simulink model "mainSim"  (Simulink 7.8)
settings: Solver=ode45  StartTime=0.0  StopTime=15  RelTol=1e-3
model workspace (MAT data in the model file):
  op_trim2 : opcond.OperatingReport (value not decoded)
values from neighbouring files (symbols this model uses):
  alt = h    [mainScript.m]
  defAilMax = 20*pi/180    (= 0.349065850399)    [mainScript.m]
  defElevMax = 25*pi/180    (= 0.436332312999)    [mainScript.m]
  defRudMax = 16*pi/180    (= 0.279252680319)    [mainScript.m]
  defThrotMax = 20    [mainScript.m]
  defTrims = [0*pi/180 -5*pi/180 0*pi/180 .5]    [mainScript.m]
  forcesReDimRefs = [Sref Sref Sref]    [mainScript.m]
  latCoeffRefs = [CY0 Cl0 Cn0]    [mainScript.m]
  latMatrix = [CYbeta CYbetaDot CYP CYR CYdeltaA CYdeltaR ... (first row only)    [mainScript.m]
  latNonDimRefs = [1 bref/(2*u0) bref/(2*u0)  bref/(2*u0) 1 1]    [mainScript.m]
  latStateRefs = [beta0 betaDot0 p0 q0 deltaA0 deltaR0]    [mainScript.m]
  longCoeffRefs = [-CD1 -CL0 CM1]    [mainScript.m]
  longMatrix = [CXu CXalpha CXalphaDot CXq CXdeltaE ... (first row only)    [mainScript.m]
  longNonDimRefs = [1/u0 1 cref/(2*u0) cref/(2*u0) 1]    [mainScript.m]
  longStateRefs = [u0 alpha0  alphaDot0 q0 deltaE0]    [mainScript.m]
  momentReDimRefs = [Sref*bref Sref*cref Sref*bref]    [mainScript.m]
  speed = v    [mainScript.m]
  Thrust = Tprop    [mainScript.m]
  Torque = QProp    [mainScript.m]
  V0 = [220 0 0]    [mainScript.m]
  Volt = V    [mainScript.m]
undefined symbols (not defined in the file or in its folder): Earth, WGS84
libraries: simulink x4, aerolibconvert2 x3, aerolibfltsims x2, aerolib6dof2 x1, aerolibatmos2 x1, aerolibtransform2 x1, aerolibasang x1, aerolibutil x1, aerolibanimutils x1
settings Model: Creator=mufasa  LastModifiedBy=atchase
settings DataIOCC: ExternalInput=getinputstruct(op_trim2)  InitialState=getstatestruct(op_trim2)  SignalLoggingSaveFormat=Dataset
settings GRTTargetCC: CombineOutputUpdateFcns=on

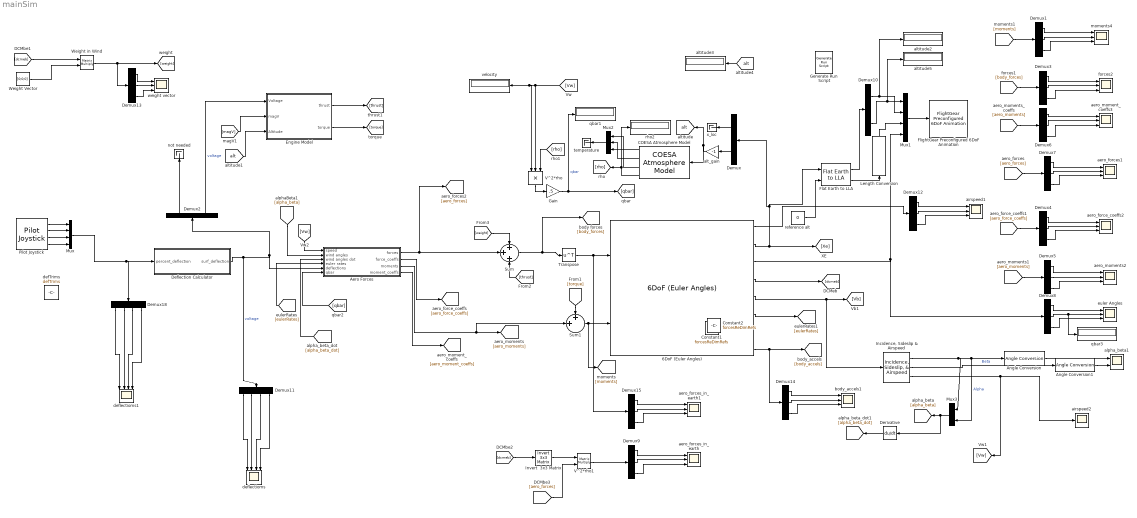
== system mainSim ==
  6DoF (Euler Angles) : aerolib6dof2/6DoF (Euler Angles)  units=English (Velocity in ft/s)  mtype=Fixed  rep=Quaternion  xme_0=X0  Vm_0=[V0(1) 0 0]  eul_0=[0 0 0]  pm_0=eulerRate0  mass_0=W  mass_e=0.5  mass_f=2.0  inertia=J  inertia_e=eye(3)  inertia_f=2*eye(3)  k_quat=1.0
  Aero Forces : Subsystem
  Angle Conversion : aerolibconvert2/Angle Conversion  IU=rad  OU=deg
  Angle Conversion1 : aerolibconvert2/Angle Conversion  IU=rad  OU=deg
  COESA Atmosphere Model : aerolibatmos2/COESA Atmosphere Model  units=English (Velocity in ft/s)  spec=1976 COESA-extended U.S. Standard Atmosphere  model=Profile  profile_var=High temperature  profile_percent=1%  profile_alt=5 km (16404 ft)  envelope_var=High temperature  envelope_percent=1%  action=Warning
  Constant1 : Constant  Value=forcesReDimRefs
  Constant2 : Constant  Value=forcesReDimRefs
  Deflection Calculator : Subsystem
  Demux : Demux  Outputs=[2 1]
  Demux{1,3..9,12..15} (12 alike) : Demux  Outputs=3
  Demux10 : Demux  Outputs=2
  Demux11 : Demux
  Demux18 : Demux
  Demux2 : Demux  Outputs=[3 1]
  Derivative : Derivative
  Engine Model : Subsystem
  Flat Earth to LLA : aerolibtransform2/Flat Earth to LLA  units=English  ptype=Earth (WGS84)  F=1/298.257223563  R=20925646.3255  LL0=[37 -121]  psi=0
  FlightGear Preconfigured 6DoF Animation : aerolibfltsims/FlightGear Preconfigured 6DoF Animation  xFlightGearVersion=v2.0  DestinationIpAddress=129.65.189.108  DestinationPort=5502  SampleTime=1/30
  Gain : Gain  Gain=.5
  Generate Run Script : aerolibfltsims/Generate Run Script  OutputFileName=runfg.bat  FlightGearBaseDirectory=C:\Program Files\FlightGear  GeometryModelName=c172p  DestinationPort=5502  AirportId=KSFO  RunwayId=10L  InitialAltitude=7224  InitialHeading=113  OffsetDistance=4.72  OffsetAzimuth=0  GenerateFile=off
  "Incidence, Sideslip & Airspeed" : aerolibasang/Incidence, Sideslip, & Airspeed
  Invert  3x3 Matrix : aerolibutil/Invert  3x3 Matrix
  Length Conversion : aerolibconvert2/Length Conversion  IU=ft  OU=m
  Mux : Mux
  Mux1 : Mux  Inputs=[1 1 1 3]
  Mux2 : Mux  Inputs=3
  Mux3 : Mux  Inputs=2
  Pilot Joystick : aerolibanimutils/Pilot Joystick  JoystickID=Joystick1  OutputConfiguration=FourAxis  SampleTime=1/30
  Sum : Sum  Inputs=+++
  Sum1 : Sum  Inputs=++|
  Transpose : Math  Operator=transpose  SaturateOnIntegerOverflow=on
  V^2*rho : Product  Inputs=3  RndMeth=Zero
  V^2*rho1 : Product  Multiplication=Matrix(*)  RndMeth=Zero
  Weight Vector : Constant  Value=[0;0;0]  VectorParams1D=off
  Weight in Wind : Product  Multiplication=Matrix(*)  RndMeth=Zero
  aero_force_coeffs2 : Scope  NumInputPorts=3
      settings: TimeRange=30  YMin=-0.5~-1~-4  YMax=0.5~1~4  SaveName=ScopeData3
  aero_forces1 : Scope  NumInputPorts=3
      settings: TimeRange=30  YMin=-2300~-1~-5000  YMax=-200~1~65000  SaveName=ScopeData4
  aero_forces_in_earth : Scope  NumInputPorts=3
      settings: TimeRange=100  YMin=-650~-1~-3515  YMax=-617.5~1~-3425  SaveName=ScopeData6
  aero_forces_in_earth1 : Scope  NumInputPorts=3
      settings: TimeRange=30  YMin=-650~-1~-3515  YMax=-617.5~1~-3425  SaveName=ScopeData11
  aero_moment_coeffs3 : Scope  NumInputPorts=3
      settings: TimeRange=30  YMin=0.309~-1~-1  YMax=0.332~1~1  SaveName=ScopeData5
  aero_moments2 : Scope  NumInputPorts=3
      settings: TimeRange=100  YMin=-1~-1~2517.5  YMax=1~1~2782.5  SaveName=ScopeData2
  airspeed1 : Scope  NumInputPorts=3
      settings: TimeRange=5  YMin=196.4~-1~-17.05  YMax=197.2~1~-16.25  SaveName=ScopeData13
  airspeed2 : Scope
      settings: TimeRange=5  YMin=213.55  YMax=213.69  SaveName=ScopeData17
  alpha_beta1 : Scope  NumInputPorts=2
      settings: TimeRange=25  YMin=-60~-1  YMax=60~1  SaveName=ScopeData16
  alt_gain : Gain  Gain=-1
  altitude2 : Display
  altitude3 : Display
  altitude5 : Display
  body_accels1 : Scope  NumInputPorts=3
      settings: TimeRange=100  YMin=-0.17~-1~-0.005  YMax=-0.156~1~0.095  SaveName=ScopeData10
  defTrims : Constant  Value=defTrims
  deflectioms : Scope  NumInputPorts=4
      settings: YMin=0.0025908~-1.1~-1~19  YMax=0.00286352~1.1~1~21  SaveName=ScopeData7
  deflectioms1 : Scope  NumInputPorts=4
      settings: TimeRange=5  YMin=-0.8~-0.01~-0.08~-1  YMax=0.6~0.08~0~1  SaveName=ScopeData14
  euler Angles : Scope  NumInputPorts=3
      settings: TimeRange=100  YMin=1.5708~2.75e-017~0.125  YMax=1.5708~8.5e-017~0.4  SaveName=ScopeData8
  forces2 : Scope  NumInputPorts=3
      settings: TimeRange=30  YMin=-119.5~-1~310.5  YMax=-116.5~1~310.69
  moments4 : Scope  NumInputPorts=3
      settings: TimeRange=30  YMin=0.309~-1~-1  YMax=0.332~1~1
  not needed : Terminator
  qbar1 : Display
  qbar3 : Display
  reference alt : Constant  Value=0
  rho2 : Display
  temperature : Terminator
  velocity : Display
  weight vector : Scope  NumInputPorts=3
      settings: TimeRange=5  YMin=-1~2517.5~5.58997e-013  YMax=1~2782.5~6.17839e-013  SaveName=ScopeData9
  x_loc : Terminator
  tag scope: alt=global
  wires:
  Pilot Joystick/1 -> Mux/1
  Pilot Joystick/2 -> Mux/2
  Pilot Joystick/3 -> Mux/3
  Pilot Joystick/4 -> Mux/4
  Deflection Calculator/1(surf_deflection) -> Demux11/1, Demux2/1, Aero Forces/5(deflections)  "voltage"
  Demux/1 -> x_loc/1
  Demux/2 -> alt_gain/1
  V^2*rho/1 -> Gain/1
  Mux/1 -> Demux18/1, Deflection Calculator/1(percent_deflection)
  reference alt/1 -> Flat Earth to LLA/2
  Mux1/1 -> FlightGear Preconfigured 6DoF Animation/1
  Flat Earth to LLA/1 -> Demux10/1
  alt_gain/1 -> [alt], COESA Atmosphere Model/1
  Demux11/1 -> deflectioms/1
  Demux11/2 -> deflectioms/2
  Demux11/3 -> deflectioms/3
  Demux11/4 -> deflectioms/4
  COESA Atmosphere Model/4 -> [rho], rho2/1
  Demux2/2 -> Engine Model/1(Voltage)  "voltage"
  Demux2/1 -> not needed/1
  [alt] -> Engine Model/3(Altitude)
  [magV] -> Engine Model/2(magV)
  Engine Model/1(thrust) -> [thrust]
  Engine Model/2(torque) -> [torque]
  Gain/1 -> [qbar], qbar1/1  "qbar"
  [alt] -> altitude3/1
  Sum1/1 -> 6DoF (Euler Angles)/2, [moments]
  [torque] -> Sum1/1
  [thrust] -> Sum/3
  Flat Earth to LLA/2 -> Length Conversion/1
  6DoF (Euler Angles)/2 -> Flat Earth to LLA/1, Demux/1, [Xe]
  6DoF (Euler Angles)/4 -> [dcmeb]
  [dcmeb] -> Weight in Wind/1
  Weight Vector/1 -> Weight in Wind/2
  Weight in Wind/1 -> [weight], Demux13/1
  Demux13/1 -> weight vector/1
  Demux13/2 -> weight vector/2
  Demux13/3 -> weight vector/3
  6DoF (Euler Angles)/3 -> Mux1/4, Demux8/1
  Length Conversion/1 -> Mux1/3
  Demux10/2 -> Mux1/1, altitude5/1
  Demux10/1 -> Mux1/2, altitude2/1
  6DoF (Euler Angles)/5 -> [Vb], "Incidence, Sideslip & Airspeed"/1
  Sum/1 -> [body_forces], Transpose/1
  6DoF (Euler Angles)/8 -> [body_accels], Demux14/1
  [qbar] -> Aero Forces/6(qbar)
  6DoF (Euler Angles)/6 -> [eulerRates]
  [eulerRates] -> Aero Forces/4(euler rates)
  [alpha_beta_dot] -> Aero Forces/3(wind angles dot)
  [alpha_beta] -> Aero Forces/2(wind angles)
  [Vw] -> Aero Forces/1(speed)
  COESA Atmosphere Model/1 -> Mux2/1
  COESA Atmosphere Model/2 -> Mux2/2
  COESA Atmosphere Model/3 -> Mux2/3
  Mux2/1 -> temperature/1
  Demux18/1 -> deflectioms1/1
  Demux18/2 -> deflectioms1/2
  Demux18/3 -> deflectioms1/3
  Demux18/4 -> deflectioms1/4
  Demux1/2 -> moments4/2
  Demux1/3 -> moments4/3
  Demux1/1 -> moments4/1
  [moments] -> Demux1/1
  [weight] -> Sum/1
  Demux3/2 -> forces2/2
  Demux3/3 -> forces2/3
  Demux3/1 -> forces2/1
  [body_forces] -> Demux3/1
  Demux4/2 -> aero_force_coeffs2/2
  Demux4/3 -> aero_force_coeffs2/3
  Demux4/1 -> aero_force_coeffs2/1
  [aero_force_coeffs] -> Demux4/1
  Demux5/2 -> aero_moments2/2
  Demux5/3 -> aero_moments2/3
  Demux5/1 -> aero_moments2/1
  [aero_moments] -> Demux5/1
  Demux6/2 -> aero_moment_coeffs3/2
  Demux6/3 -> aero_moment_coeffs3/3
  Demux6/1 -> aero_moment_coeffs3/1
  [aero_moments] -> Demux6/1
  Demux7/2 -> aero_forces1/2
  Demux7/3 -> aero_forces1/3
  Demux7/1 -> aero_forces1/1
  [aero_forces] -> Demux7/1
  Demux12/2 -> airspeed1/2
  Demux12/3 -> airspeed1/3
  Demux12/1 -> airspeed1/1
  6DoF (Euler Angles)/1 -> Demux12/1
  "Incidence, Sideslip & Airspeed"/1 -> Mux3/1, Mux3/2, Angle Conversion/1  "Alpha"
  "Incidence, Sideslip & Airspeed"/2 -> Angle Conversion1/1  "Beta"
  Mux3/1 -> [alpha_beta], Derivative/1
  Derivative/1 -> [alpha_beta_dot]
  "Incidence, Sideslip & Airspeed"/3 -> airspeed2/1, [Vw]
  [Vw] -> V^2*rho/2, velocity/1, V^2*rho/1
  [rho] -> V^2*rho/3
  Angle Conversion/1 -> alpha_beta1/1
  Angle Conversion1/1 -> alpha_beta1/2
  Demux8/2 -> euler Angles/2, qbar3/1
  Demux8/3 -> euler Angles/3
  Demux8/1 -> euler Angles/1
  [dcmeb] -> Invert  3x3 Matrix/1
  Invert  3x3 Matrix/1 -> V^2*rho1/1
  [aero_forces] -> V^2*rho1/2
  Demux9/2 -> aero_forces_in_earth/2
  Demux9/3 -> aero_forces_in_earth/3
  Demux9/1 -> aero_forces_in_earth/1
  V^2*rho1/1 -> Demux9/1
  Demux14/2 -> body_accels1/2
  Demux14/3 -> body_accels1/3
  Demux14/1 -> body_accels1/1
  Demux15/2 -> aero_forces_in_earth1/2
  Demux15/3 -> aero_forces_in_earth1/3
  Demux15/1 -> aero_forces_in_earth1/1
  Aero Forces/2(force_coeffs) -> [aero_force_coeffs]
  Aero Forces/4(moment_coeffs) -> [aero_moment_coeffs]
  Aero Forces/1(forces) -> [aero_forces], Sum/2
  Aero Forces/3(moments) -> [aero_moments], Sum1/2
  Transpose/1 -> 6DoF (Euler Angles)/1, Demux15/1

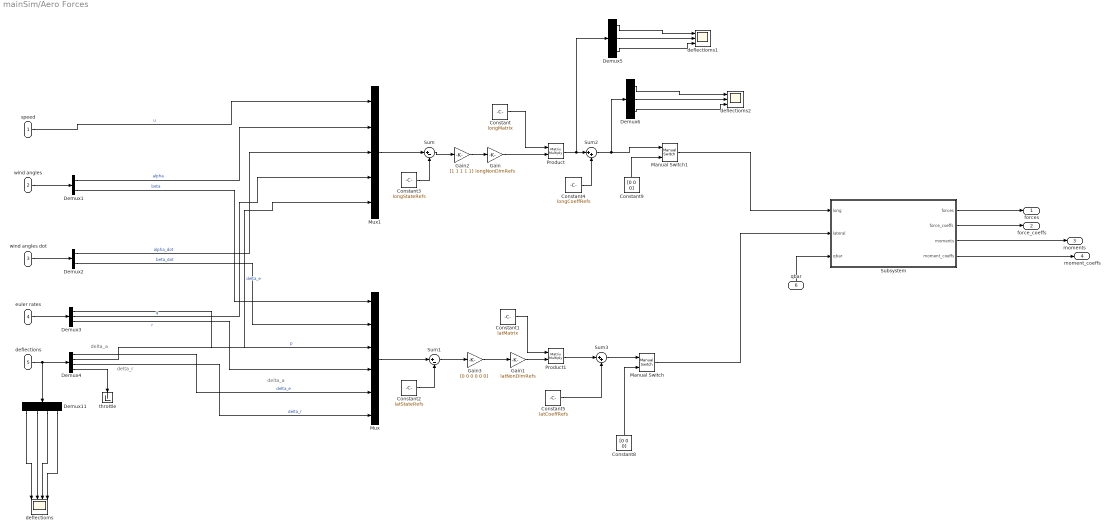
== system mainSim/Aero Forces ==
  note: delta_a
  note: delta_r
  note: delta_a
  speed : Inport
  wind angles : Inport  Port=2
  wind angles dot : Inport  Port=3
  euler rates : Inport  Port=4
  deflections : Inport  Port=5
  qbar : Inport  Port=6
  Constant : Constant  Value=longMatrix
  Constant1 : Constant  Value=latMatrix
  Constant2 : Constant  Value=latStateRefs
  Constant3 : Constant  Value=longStateRefs
  Constant4 : Constant  Value=longCoeffRefs
  Constant5 : Constant  Value=latCoeffRefs
  Constant8 : Constant  Value=[0 0 0]
  Constant9 : Constant  Value=[0 0 0]
  Demux1 : Demux  Outputs=2
  Demux11 : Demux
  Demux2 : Demux  Outputs=2
  Demux3 : Demux  Outputs=3
  Demux4 : Demux
  Demux5 : Demux  Outputs=3
  Demux6 : Demux  Outputs=3
  Gain : Gain  Gain=longNonDimRefs
  Gain1 : Gain  Gain=latNonDimRefs
  Gain2 : Gain  Gain=[1 1 1 1 1]
  Gain3 : Gain  Gain=[0 0 0 0 0 0]
  Manual Switch : simulink/Signal Routing/Manual Switch  sw=1  action=0  varsize=off
  Manual Switch1 : simulink/Signal Routing/Manual Switch  sw=1  action=0  varsize=off
  Mux : Mux  Inputs=6
  Mux1 : Mux  Inputs=5
  Product : Product  Multiplication=Matrix(*)  RndMeth=Zero
  Product1 : Product  Multiplication=Matrix(*)  RndMeth=Zero
  Subsystem : Subsystem
  Sum : Sum  Inputs=|+-
  Sum1 : Sum  Inputs=|+-
  Sum2 : Sum  Inputs=|++
  Sum3 : Sum  Inputs=|++
  deflectioms : Scope  NumInputPorts=4
      settings: YMin=0.0025908~-1.1~-1~19  YMax=0.00286352~1.1~1~21  SaveName=ScopeData15
  deflectioms1 : Scope  NumInputPorts=3
      settings: TimeRange=200  YMin=0.0025908~-1.1~-1  YMax=0.00286352~1.1~1  SaveName=ScopeData12
  deflectioms2 : Scope  NumInputPorts=3
      settings: TimeRange=200  YMin=0.0025908~-1.1~-1  YMax=0.00286352~1.1~1  SaveName=ScopeData18
  throttle : Terminator
  forces : Outport
  force_coeffs : Outport  Port=2
  moments : Outport  Port=3
  moment_coeffs : Outport  Port=4
  wires:
  speed/1 -> Mux1/1  "u"
  wind angles/1 -> Demux1/1
  wind angles dot/1 -> Demux2/1
  euler rates/1 -> Demux3/1
  deflections/1 -> Demux11/1, Demux4/1
  Demux1/1 -> Mux1/2  "alpha"
  Demux2/1 -> Mux1/3  "alpha_dot"
  Demux11/1 -> deflectioms/1
  Demux11/2 -> deflectioms/2
  Demux11/3 -> deflectioms/3
  Demux11/4 -> deflectioms/4
  Demux4/4 -> throttle/1
  Demux4/2 -> Mux1/5  "delta_e"
  Demux3/2 -> Mux1/4  "q"
  Demux1/2 -> Mux/1  "beta"
  Demux2/2 -> Mux/2  "beta_dot"
  Demux3/1 -> Mux/3  "p"
  Demux3/3 -> Mux/4  "r"
  Demux4/3 -> Mux/6  "delta_r"
  Demux4/1 -> Mux/5  "delta_e"
  Constant/1 -> Product/1
  Constant1/1 -> Product1/1
  Mux1/1 -> Sum/1
  Mux/1 -> Sum1/1
  Sum1/1 -> Gain3/1
  Constant2/1 -> Sum1/2
  Constant3/1 -> Sum/2
  Sum/1 -> Gain2/1
  Product/1 -> Sum2/1, Demux5/1
  Product1/1 -> Sum3/1
  Constant4/1 -> Sum2/2
  Constant5/1 -> Sum3/2
  Gain/1 -> Product/2
  Gain1/1 -> Product1/2
  Sum2/1 -> Manual Switch1/1, Demux6/1
  Sum3/1 -> Manual Switch/1
  Constant8/1 -> Manual Switch/2
  Constant9/1 -> Manual Switch1/2
  Manual Switch1/1 -> Subsystem/1(long)
  Manual Switch/1 -> Subsystem/2(lateral)
  qbar/1 -> Subsystem/3(qbar)
  Subsystem/1(forces) -> forces/1
  Subsystem/2(force_coeffs) -> force_coeffs/1
  Demux5/1 -> deflectioms1/1
  Demux5/2 -> deflectioms1/2
  Demux5/3 -> deflectioms1/3
  Demux6/1 -> deflectioms2/1
  Demux6/2 -> deflectioms2/2
  Demux6/3 -> deflectioms2/3
  Gain2/1 -> Gain/1
  Gain3/1 -> Gain1/1
  Subsystem/3(moments) -> moments/1
  Subsystem/4(moment_coeffs) -> moment_coeffs/1

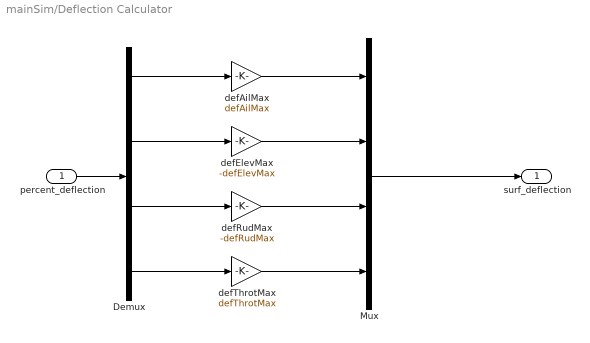
== system mainSim/Deflection Calculator ==
  percent_deflection : Inport
  Demux : Demux
  Mux : Mux
  defAilMax : Gain  Gain=defAilMax
  defElevMax : Gain  Gain=-defElevMax
  defRudMax : Gain  Gain=-defRudMax
  defThrotMax : Gain  Gain=defThrotMax
  surf_deflection : Outport
  wires:
  percent_deflection/1 -> Demux/1
  Demux/1 -> defAilMax/1
  Demux/2 -> defElevMax/1
  Demux/3 -> defRudMax/1
  Demux/4 -> defThrotMax/1
  Mux/1 -> surf_deflection/1
  defAilMax/1 -> Mux/1
  defElevMax/1 -> Mux/2
  defRudMax/1 -> Mux/3
  defThrotMax/1 -> Mux/4

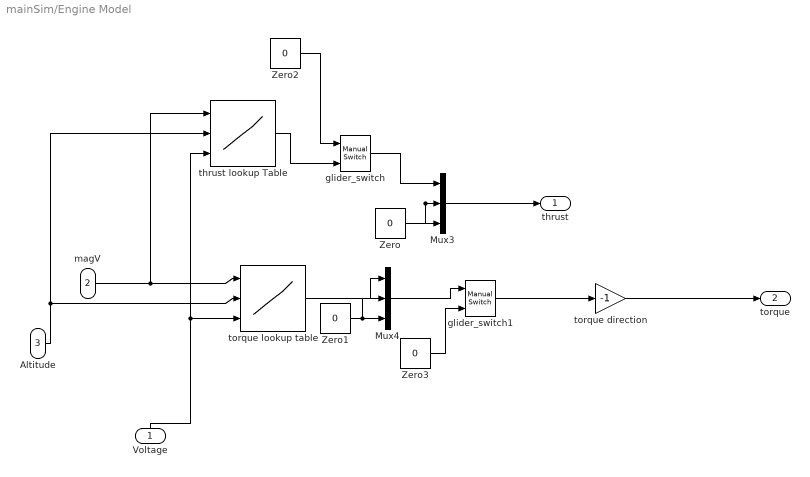
== system mainSim/Engine Model ==
  Voltage : Inport
  magV : Inport  Port=2
  Altitude : Inport  Port=3
  Mux3 : Mux  Inputs=3
  Mux4 : Mux  Inputs=3
  Zero{,1..3} (4 alike) : Constant  Value=0
  glider_switch : simulink/Signal Routing/Manual Switch  sw=1  action=0  varsize=off
  glider_switch1 : simulink/Signal Routing/Manual Switch  sw=0  action=0  varsize=off
  thrust lookup Table : Lookup_n-D  NumberOfTableDimensions=3  BreakpointsForDimension1=speed  BreakpointsForDimension2=alt  BreakpointsForDimension3=Volt  Table=Thrust  RndMeth=Simplest  InputSameDT=on
  torque direction : Gain  Gain=-1
  torque lookup table : Lookup_n-D  NumberOfTableDimensions=3  BreakpointsForDimension1=speed  BreakpointsForDimension2=alt  BreakpointsForDimension3=Volt  Table=Torque  RndMeth=Simplest  InputSameDT=on
  thrust : Outport
  torque : Outport  Port=2
  wires:
  Zero/1 -> Mux3/3, Mux3/2
  torque lookup table/1 -> Mux4/1
  Zero1/1 -> Mux4/2, Mux4/3
  Zero2/1 -> glider_switch/1
  glider_switch/1 -> Mux3/1
  thrust lookup Table/1 -> glider_switch/2
  glider_switch1/1 -> torque direction/1
  Mux4/1 -> glider_switch1/1
  Zero3/1 -> glider_switch1/2
  Voltage/1 -> torque lookup table/3, thrust lookup Table/3
  Altitude/1 -> torque lookup table/2, thrust lookup Table/2
  magV/1 -> torque lookup table/1, thrust lookup Table/1
  torque direction/1 -> torque/1
  Mux3/1 -> thrust/1

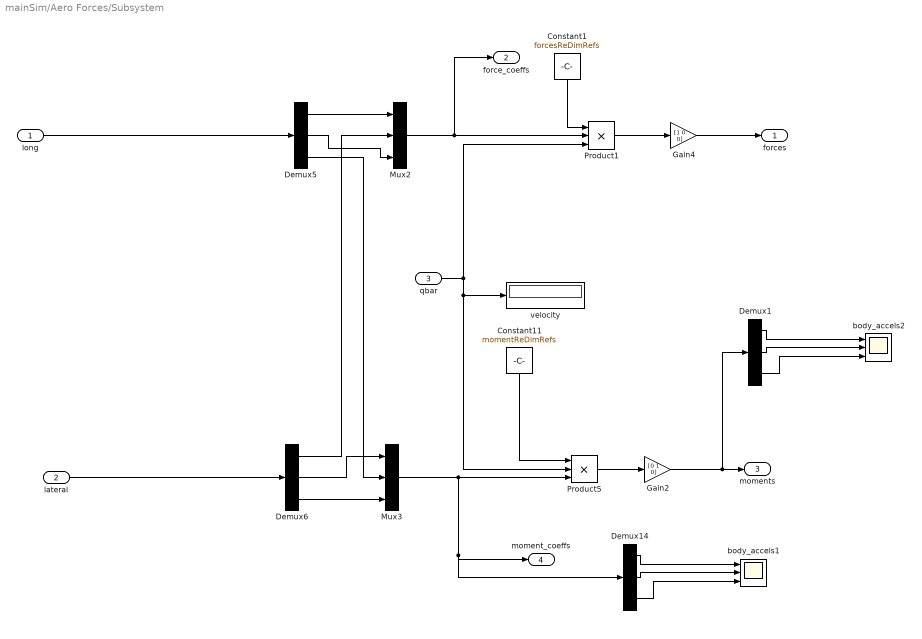
== system mainSim/Aero Forces/Subsystem ==
  long : Inport
  lateral : Inport  Port=2
  qbar : Inport  Port=3
  Constant1 : Constant  Value=forcesReDimRefs
  Constant11 : Constant  Value=momentReDimRefs
  Demux{1,5..6,14} (4 alike) : Demux  Outputs=3
  Gain2 : Gain  Gain=[0 1 0]
  Gain4 : Gain  Gain=[1 0 0]
  Mux2 : Mux  Inputs=3
  Mux3 : Mux  Inputs=3
  Product1 : Product  Inputs=3  RndMeth=Zero
  Product5 : Product  Inputs=3  RndMeth=Zero
  body_accels1 : Scope  NumInputPorts=3
      settings: TimeRange=100  YMin=-0.17~-1~-0.005  YMax=-0.156~1~0.095  SaveName=ScopeData19
  body_accels2 : Scope  NumInputPorts=3
      settings: TimeRange=100  YMin=-0.17~-1~-0.005  YMax=-0.156~1~0.095  SaveName=ScopeData20
  velocity : Display
  forces : Outport
  force_coeffs : Outport  Port=2
  moments : Outport  Port=3
  moment_coeffs : Outport  Port=4
  wires:
  Demux6/1 -> Mux2/2
  Demux6/2 -> Mux3/1
  Demux6/3 -> Mux3/3
  Demux5/3 -> Mux3/2
  Mux3/1 -> Product5/3, moment_coeffs/1, Demux14/1
  Demux5/2 -> Mux2/3
  Demux5/1 -> Mux2/1
  Constant11/1 -> Product5/1
  Mux2/1 -> force_coeffs/1, Product1/2
  long/1 -> Demux5/1
  lateral/1 -> Demux6/1
  Gain4/1 -> forces/1
  qbar/1 -> Product5/2, velocity/1, Product1/3
  Constant1/1 -> Product1/1
  Product1/1 -> Gain4/1
  Gain2/1 -> moments/1, Demux1/1
  Product5/1 -> Gain2/1
  Demux14/2 -> body_accels1/2
  Demux14/3 -> body_accels1/3
  Demux14/1 -> body_accels1/1
  Demux1/2 -> body_accels2/2
  Demux1/3 -> body_accels2/3
  Demux1/1 -> body_accels2/1
